simulink model "Complementary_filter"  (R2025b)
settings: Solver=ode4  StartTime=0.0  StopTime=50  FixedStep=0.002  RelTol=1e-3
values from neighbouring files (symbols this model uses):
  fa = 2*pi*2    (= 12.5663706144)    [Parameters.m]
  fg = 2*pi*8    (= 50.2654824574)    [Parameters.m]
  kda = 0.27*ktha    (= 0.0005184)    [Parameters.m]
  ki = fc^2    (= 0.394784176044)    [Parameters.m]
  kp = 2.0*0.707*fc    (= 0.888442402435)    [Parameters.m]
  kpa = ktha    (= 0.00192)    [Parameters.m]
settings Model: Creator=yfari  LastModifiedBy=yfari
settings OptimizationCC: ReuseModelBlockBuffer=off
settings DebuggingCC: UnconnectedInputMsg=warning  UnconnectedOutputMsg=warning  UnconnectedLineMsg=warning
settings ModelReferenceCC: EnableRefExpFcnMdlSchedulingChecks=on
settings RTWCC: GPUComputeCapability=3.5  DLArmComputeVersion=19.05

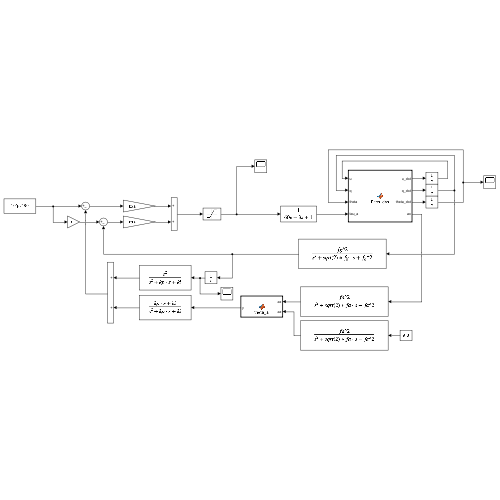
[thumbnail: Simulink's stored preview of the top-level diagram]
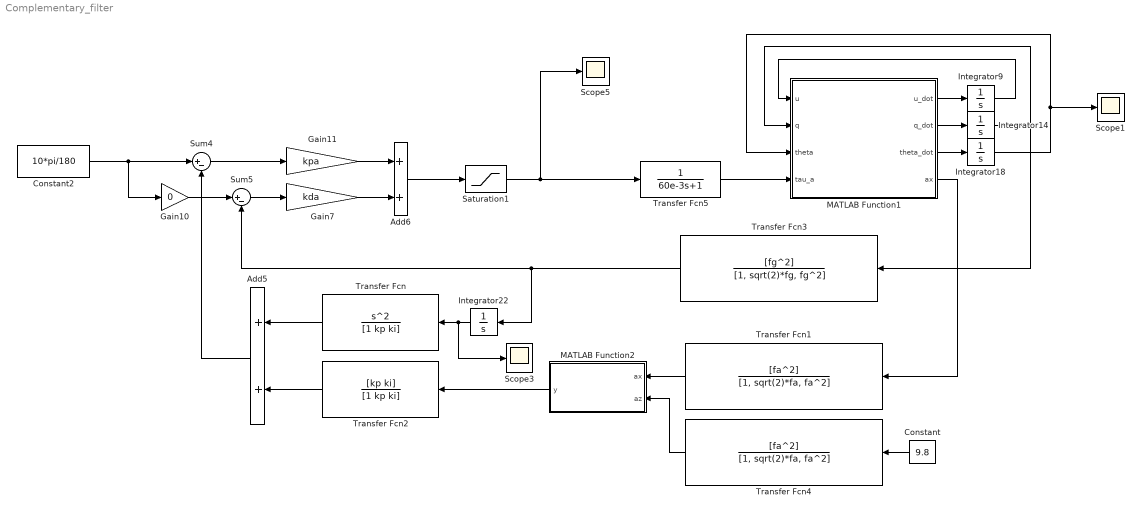
== system Complementary_filter ==
  Add5 : Sum
  Add6 : Sum
  Constant : Constant  Value=9.8
  Constant2 : Constant  Value=10*pi/180
  Gain10 : Gain  Gain=0
  Gain11 : Gain  Gain=kpa
  Gain7 : Gain  Gain=kda
  Integrator{9,14,18,22} (4 alike) : Integrator
  MATLAB Function1 : MATLAB Function  TreatAsAtomicUnit=on
  MATLAB Function2 : MATLAB Function  TreatAsAtomicUnit=on
  Saturation1 : Saturate  UpperLimit=0.002  LowerLimit=-0.002
  Scope1 : Scope
      settings: ActiveDisplayYMinimum=-1  ActiveDisplayYMaximum=1
  Scope3 : Scope
      settings: ActiveDisplayYMinimum=-0.78342  ActiveDisplayYMaximum=0.10035  DataLoggingVariableName=ScopeData4
  Scope5 : Scope
      settings: ActiveDisplayYMinimum=-0.00184  ActiveDisplayYMaximum=0.0017
  Sum4 : Sum  Inputs=|+-
  Sum5 : Sum  Inputs=|+-
  Transfer Fcn : TransferFcn  Numerator=[1 0 0]  Denominator=[1 kp ki]
  Transfer Fcn1 : TransferFcn  Numerator=[fa^2]  Denominator=[1, sqrt(2)*fa, fa^2]
  Transfer Fcn2 : TransferFcn  Numerator=[kp ki]  Denominator=[1 kp ki]
  Transfer Fcn3 : TransferFcn  Numerator=[fg^2]  Denominator=[1, sqrt(2)*fg, fg^2]
  Transfer Fcn4 : TransferFcn  Numerator=[fa^2]  Denominator=[1, sqrt(2)*fa, fa^2]
  Transfer Fcn5 : TransferFcn  Denominator=[60e-3 1]
  wires:
  Gain7/1 -> Add6/2
  MATLAB Function2/1(y) -> Transfer Fcn2/1
  Transfer Fcn2/1 -> Add5/2
  Transfer Fcn3/1 -> Sum5/2, Integrator22/1
  Gain11/1 -> Add6/1
  Gain10/1 -> Sum5/1
  Saturation1/1 -> Scope5/1, Transfer Fcn5/1
  Add5/1 -> Sum4/2
  Transfer Fcn/1 -> Add5/1
  MATLAB Function1/2(q_dot) -> Integrator14/1
  Constant/1 -> Transfer Fcn4/1
  Integrator22/1 -> Scope3/1, Transfer Fcn/1
  Integrator18/1 -> Scope1/1, MATLAB Function1/3(theta)
  MATLAB Function1/1(u_dot) -> Integrator9/1
  Transfer Fcn4/1 -> MATLAB Function2/2(az)
  Add6/1 -> Saturation1/1
  Sum4/1 -> Gain11/1
  Integrator9/1 -> MATLAB Function1/1(u)
  Sum5/1 -> Gain7/1
  MATLAB Function1/3(theta_dot) -> Integrator18/1
  Transfer Fcn1/1 -> MATLAB Function2/1(ax)
  Transfer Fcn5/1 -> MATLAB Function1/4(tau_a)
  Integrator14/1 -> Transfer Fcn3/1, MATLAB Function1/2(q)
  MATLAB Function1/4(ax) -> Transfer Fcn1/1
  Constant2/1 -> Gain10/1, Sum4/1

== matlab function Complementary_filter/MATLAB Function1 ==
  data: u input; u_dot output; q input; theta input; q_dot output; theta_dot output; tau_a input; ax output
function [u_dot, q_dot, theta_dot, ax] = Pitch_dyn(u, q, theta, tau_a)

m = 23.5*(10^-3);
K = 22.3*(10^-3);
K_q = 0.008*(10^-3);
K_r = 0.065*(10^-3);
I_yy = 56000*(10^-3)*(10^-3)^2;
T = 60*10^-3;
g = 9.81;

zd = 15*10^-3;
zb = 60*10^-3 + zd;
X_u = -K;
X_q = -K*zd;
M_u = X_q;
M_q = -K_q - K*zd^2;
X_hat_u = X_u/m;
M_hat_q = M_q/I_yy;
M_hat_u = M_u/I_yy;
X_hat_q = X_q/m;
%% %%
u_dot = X_hat_u*u + X_hat_q*q + g*theta;
q_dot = M_hat_u*u + M_hat_q*q + tau_a/I_yy;
theta_dot = q;
ax = - X_hat_u*u - X_hat_q*q;
end

== matlab function Complementary_filter/MATLAB Function2 ==
  data: ax input; y output; az input
function y = theta_a(ax,az)

y = atan2(ax,az);
end
